simulink library "halin"  (R2021b)
settings: Solver=VariableStepAuto  StartTime=0.0  StopTime=10.0  RelTol=1e-3
undefined symbols (not defined in the file): KHAL_CAN1ABM1E2E_flg, KHAL_CAN1EPB1E2E_flg, KHAL_CAN1EPS1E2E_flg, KHAL_CAN1ESC1E2E_flg, KHAL_CAN1ESC5E2E_flg, KHAL_CAN3BMS1E2E_flg, KHAL_CAN3BMS6E2E_flg, KHAL_CAN3CCU1E2E_flg, KHAL_CAN3CCU2E2E_flg, KHAL_CAN3MCUBF1E2E_flg, KHAL_CAN3MCUBR1E2E_flg, KHAL_CAN3MCUNF1E2E_flg, KHAL_CAN3MCUNR1E2E_flg, KHAL_CAN3Shifter1E2E_flg, KHAL_CAN3Shifter2E2E_flg, KHAL_CAN6FCM2E2E_flg, KHAL_CAN6FCM4E2E_flg, TRUE
libraries: simulink x791, FVT_lib x214, hcu_lib x58
(part 23 of 25)

== system halin/HAL_IN/CAN3/MCU_N_R2/RrCoolanttempReqNidec ==
  Rr_CoolanttempReq_Nidec : Inport
  UnitConverter : DataTypeConversion  OutDataTypeStr=uint16
  convert_in : FVT_lib/hal/convert_in  gain=1  offset=-40
  VHAL_RrCoolanttempReqNidec_cnt : Outport
  wires:
  convert_in/1 -> VHAL_RrCoolanttempReqNidec_cnt/1
  UnitConverter/1 -> convert_in/1
  Rr_CoolanttempReq_Nidec/1 -> UnitConverter/1

== system halin/HAL_IN/CAN3/MCU_N_R2/RrEOPSpdSetNidec ==
  Rr_EOP_SpdSet_Nidec : Inport
  UnitConverter : DataTypeConversion  OutDataTypeStr=uint16
  VHAL_RrEOPSpdSetNidec_rpm : Outport
  wires:
  UnitConverter/1 -> VHAL_RrEOPSpdSetNidec_rpm/1
  Rr_EOP_SpdSet_Nidec/1 -> UnitConverter/1

== system halin/HAL_IN/CAN3/MCU_N_R2/RrFailcode1Nidec ==
  Rr_Failcode1_Nidec : Inport
  UnitConverter : DataTypeConversion  OutDataTypeStr=uint8
  VHAL_RrFailcode1Nidec_enum : Outport
  wires:
  UnitConverter/1 -> VHAL_RrFailcode1Nidec_enum/1
  Rr_Failcode1_Nidec/1 -> UnitConverter/1

== system halin/HAL_IN/CAN3/MCU_N_R2/RrFailcode2Nidec ==
  Rr_Failcode2_Nidec : Inport
  UnitConverter : DataTypeConversion  OutDataTypeStr=uint8
  VHAL_RrFailcode2Nidec_enum : Outport
  wires:
  UnitConverter/1 -> VHAL_RrFailcode2Nidec_enum/1
  Rr_Failcode2_Nidec/1 -> UnitConverter/1

== system halin/HAL_IN/CAN3/MCU_N_R2/RrFailcodehistory1Nidec ==
  Rr_Failcodehistory1_Nidec : Inport
  UnitConverter : DataTypeConversion  OutDataTypeStr=uint8
  VHAL_RrFailcodehistory1Nidec_enum : Outport
  wires:
  UnitConverter/1 -> VHAL_RrFailcodehistory1Nidec_enum/1
  Rr_Failcodehistory1_Nidec/1 -> UnitConverter/1

== system halin/HAL_IN/CAN3/MCU_N_R2/RrFailcodehistory2Nidec ==
  Rr_Failcodehistory2_Nidec : Inport
  UnitConverter : DataTypeConversion  OutDataTypeStr=uint8
  VHAL_RrFailcodehistory2Nidec_enum : Outport
  wires:
  UnitConverter/1 -> VHAL_RrFailcodehistory2Nidec_enum/1
  Rr_Failcodehistory2_Nidec/1 -> UnitConverter/1

== system halin/HAL_IN/CAN3/MCU_N_R2/RrLLCTempNidec ==
  Rr_LLCTemp_Nidec : Inport
  UnitConverter : DataTypeConversion  OutDataTypeStr=uint16
  convert_in : FVT_lib/hal/convert_in  gain=1  offset=-40
  VHAL_RrLLCTempNidec_C : Outport
  wires:
  convert_in/1 -> VHAL_RrLLCTempNidec_C/1
  UnitConverter/1 -> convert_in/1
  Rr_LLCTemp_Nidec/1 -> UnitConverter/1

== system halin/HAL_IN/CAN3/MCU_N_R2/RrLLCflowReqNidec ==
  Rr_LLCflowReq_Nidec : Inport
  UnitConverter : DataTypeConversion  OutDataTypeStr=uint8
  convert_in : FVT_lib/hal/convert_in  gain=0.25  offset=0
  VHAL_RrLLCflowReqNidec_Lpmin : Outport
  wires:
  convert_in/1 -> VHAL_RrLLCflowReqNidec_Lpmin/1
  UnitConverter/1 -> convert_in/1
  Rr_LLCflowReq_Nidec/1 -> UnitConverter/1

== system halin/HAL_IN/CAN3/MCU_N_R2/RrMCUTempWarnNidec ==
  Rr_MCUTempWarn_Nidec : Inport
  UnitConverter : DataTypeConversion  OutDataTypeStr=uint8
  VHAL_RrMCUTempWarnNidec_enum : Outport
  wires:
  UnitConverter/1 -> VHAL_RrMCUTempWarnNidec_enum/1
  Rr_MCUTempWarn_Nidec/1 -> UnitConverter/1

== system halin/HAL_IN/CAN3/MCU_N_R2/RrTMTempWarnNidec ==
  Rr_TMTempWarn_Nidec : Inport
  UnitConverter : DataTypeConversion  OutDataTypeStr=uint8
  VHAL_RrTMTempWarnNidec_enum : Outport
  wires:
  UnitConverter/1 -> VHAL_RrTMTempWarnNidec_enum/1
  Rr_TMTempWarn_Nidec/1 -> UnitConverter/1

== system halin/HAL_IN/CAN3/MCU_N_R3/RrMCU3HWVerNidec ==
  Rr_MCU3_HW_Ver_Nidec : Inport
  UnitConverter : DataTypeConversion  OutDataTypeStr=uint16
  VHAL_RrMCU3HWVerNidec_enum : Outport
  wires:
  UnitConverter/1 -> VHAL_RrMCU3HWVerNidec_enum/1
  Rr_MCU3_HW_Ver_Nidec/1 -> UnitConverter/1

== system halin/HAL_IN/CAN3/MCU_N_R3/RrMCU3SWVerNidec ==
  Rr_MCU3_SW_Ver_Nidec : Inport
  UnitConverter : DataTypeConversion  OutDataTypeStr=uint16
  VHAL_RrMCU3SWVerNidec_enum : Outport
  wires:
  UnitConverter/1 -> VHAL_RrMCU3SWVerNidec_enum/1
  Rr_MCU3_SW_Ver_Nidec/1 -> UnitConverter/1

== system halin/HAL_IN/CAN3/Shifter1/ShifterCRC8 ==
  Shifter_CRC8 : Inport
  UnitConverter : DataTypeConversion  OutDataTypeStr=uint8
  VHAL_ShifterCRC8_enum : Outport
  wires:
  UnitConverter/1 -> VHAL_ShifterCRC8_enum/1
  Shifter_CRC8/1 -> UnitConverter/1

== system halin/HAL_IN/CAN3/Shifter1/ShifterFailsta ==
  Shifter_Fail_sta : Inport
  UnitConverter : DataTypeConversion  OutDataTypeStr=uint8
  VHAL_ShifterFailsta_enum : Outport
  wires:
  UnitConverter/1 -> VHAL_ShifterFailsta_enum/1
  Shifter_Fail_sta/1 -> UnitConverter/1

== system halin/HAL_IN/CAN3/Shifter1/ShifterHandleCmd ==
  Shifter_Handle_Cmd : Inport
  UnitConverter : DataTypeConversion  OutDataTypeStr=uint8
  VHAL_ShifterHandleCmd_enum : Outport
  wires:
  UnitConverter/1 -> VHAL_ShifterHandleCmd_enum/1
  Shifter_Handle_Cmd/1 -> UnitConverter/1

== system halin/HAL_IN/CAN3/Shifter1/ShifterRC ==
  Shifter_RC : Inport
  UnitConverter : DataTypeConversion  OutDataTypeStr=uint8
  VHAL_ShifterRC_enum : Outport
  wires:
  UnitConverter/1 -> VHAL_ShifterRC_enum/1
  Shifter_RC/1 -> UnitConverter/1

== system halin/HAL_IN/CAN3/Shifter2/CSW2DimSwSta ==
  CSW2_DimSw_Sta : Inport
  UnitConverter : DataTypeConversion  OutDataTypeStr=uint8
  VHAL_CSW2DimSwSta_flg : Outport
  wires:
  UnitConverter/1 -> VHAL_CSW2DimSwSta_flg/1
  CSW2_DimSw_Sta/1 -> UnitConverter/1

== system halin/HAL_IN/CAN3/Shifter2/CSW2FWasSwSta ==
  CSW2_FWasSw_Sta : Inport
  UnitConverter : DataTypeConversion  OutDataTypeStr=uint8
  VHAL_CSW2FWasSwSta_enum : Outport
  wires:
  UnitConverter/1 -> VHAL_CSW2FWasSwSta_enum/1
  CSW2_FWasSw_Sta/1 -> UnitConverter/1

== system halin/HAL_IN/CAN3/Shifter2/CSW2FWipSwSta ==
  CSW2_FWipSw_Sta : Inport
  UnitConverter : DataTypeConversion  OutDataTypeStr=uint8
  VHAL_CSW2FWipSwSta_enum : Outport
  wires:
  UnitConverter/1 -> VHAL_CSW2FWipSwSta_enum/1
  CSW2_FWipSw_Sta/1 -> UnitConverter/1

== system halin/HAL_IN/CAN3/Shifter2/CSW2PassSWSta ==
  CSW2_PassSW_Sta : Inport
  UnitConverter : DataTypeConversion  OutDataTypeStr=uint8
  VHAL_CSW2PassSWSta_flg : Outport
  wires:
  UnitConverter/1 -> VHAL_CSW2PassSWSta_flg/1
  CSW2_PassSW_Sta/1 -> UnitConverter/1

== system halin/HAL_IN/CAN3/Shifter2/CSW2RWipWasSwSta ==
  CSW2_RWipWasSw_Sta : Inport
  UnitConverter : DataTypeConversion  OutDataTypeStr=uint8
  VHAL_CSW2RWipWasSwSta_enum : Outport
  wires:
  UnitConverter/1 -> VHAL_CSW2RWipWasSwSta_enum/1
  CSW2_RWipWasSw_Sta/1 -> UnitConverter/1

== system halin/HAL_IN/CAN3/Shifter2/CSW2TurnSwSta ==
  CSW2_TurnSw_Sta : Inport
  UnitConverter : DataTypeConversion  OutDataTypeStr=uint8
  VHAL_CSW2TurnSwSta_enum : Outport
  wires:
  UnitConverter/1 -> VHAL_CSW2TurnSwSta_enum/1
  CSW2_TurnSw_Sta/1 -> UnitConverter/1

== system halin/HAL_IN/CAN4/BodyZone_DR1/BDDSEATAntiSta ==
  BD_DSEAT_Anti_Sta : Inport
  UnitConverter : DataTypeConversion  OutDataTypeStr=uint8
  VHAL_BDDSEATAntiSta_flg : Outport
  wires:
  UnitConverter/1 -> VHAL_BDDSEATAntiSta_flg/1
  BD_DSEAT_Anti_Sta/1 -> UnitConverter/1

== system halin/HAL_IN/CAN4/BodyZone_DR1/BDDSEATEntryFunSta ==
  BD_DSEAT_EntryFun_Sta : Inport
  UnitConverter : DataTypeConversion  OutDataTypeStr=uint8
  VHAL_BDDSEATEntryFunSta_flg : Outport
  wires:
  UnitConverter/1 -> VHAL_BDDSEATEntryFunSta_flg/1
  BD_DSEAT_EntryFun_Sta/1 -> UnitConverter/1

== system halin/HAL_IN/CAN4/BodyZone_DR1/BDDSEATErrorSta ==
  BD_DSEAT_Error_Sta : Inport
  UnitConverter : DataTypeConversion  OutDataTypeStr=uint8
  VHAL_BDDSEATErrorSta_flg : Outport
  wires:
  UnitConverter/1 -> VHAL_BDDSEATErrorSta_flg/1
  BD_DSEAT_Error_Sta/1 -> UnitConverter/1

== system halin/HAL_IN/CAN4/BodyZone_DR1/BDDSEATMemSetSta ==
  BD_DSEAT_MemSet_Sta : Inport
  UnitConverter : DataTypeConversion  OutDataTypeStr=uint8
  VHAL_BDDSEATMemSetSta_enum : Outport
  wires:
  UnitConverter/1 -> VHAL_BDDSEATMemSetSta_enum/1
  BD_DSEAT_MemSet_Sta/1 -> UnitConverter/1

== system halin/HAL_IN/CAN4/BodyZone_DR1/BDDSEATModeSta ==
  BD_DSEAT_Mode_Sta : Inport
  UnitConverter : DataTypeConversion  OutDataTypeStr=uint8
  VHAL_BDDSEATModeSta_enum : Outport
  wires:
  UnitConverter/1 -> VHAL_BDDSEATModeSta_enum/1
  BD_DSEAT_Mode_Sta/1 -> UnitConverter/1

== system halin/HAL_IN/CAN4/BodyZone_DR1/BDDSEATVentSta ==
  BD_DSEAT_Vent_Sta : Inport
  UnitConverter : DataTypeConversion  OutDataTypeStr=uint8
  VHAL_BDDSEATVentSta_enum : Outport
  wires:
  UnitConverter/1 -> VHAL_BDDSEATVentSta_enum/1
  BD_DSEAT_Vent_Sta/1 -> UnitConverter/1

== system halin/HAL_IN/CAN4/BodyZone_DR1/BDDSEATheaterSta ==
  BD_DSEAT_heater_Sta : Inport
  UnitConverter : DataTypeConversion  OutDataTypeStr=uint8
  VHAL_BDDSEATheaterSta_enum : Outport
  wires:
  UnitConverter/1 -> VHAL_BDDSEATheaterSta_enum/1
  BD_DSEAT_heater_Sta/1 -> UnitConverter/1

== system halin/HAL_IN/CAN4/BodyZone_DR2/BDAPMWinFOpenedSta ==
  BD_APM_WinFOpened_Sta : Inport
  UnitConverter : DataTypeConversion  OutDataTypeStr=uint8
  VHAL_BDAPMWinFOpenedSta_pct : Outport
  wires:
  UnitConverter/1 -> VHAL_BDAPMWinFOpenedSta_pct/1
  BD_APM_WinFOpened_Sta/1 -> UnitConverter/1

== system halin/HAL_IN/CAN4/BodyZone_DR2/BDAPMWinROpenedSta ==
  BD_APM_WinROpened_Sta : Inport
  UnitConverter : DataTypeConversion  OutDataTypeStr=uint8
  VHAL_BDAPMWinROpenedSta_pct : Outport
  wires:
  UnitConverter/1 -> VHAL_BDAPMWinROpenedSta_pct/1
  BD_APM_WinROpened_Sta/1 -> UnitConverter/1

== system halin/HAL_IN/CAN4/BodyZone_DR2/BDDoorFHandleCloseSta ==
  BD_Door_FHandleClose_Sta : Inport
  UnitConverter : DataTypeConversion  OutDataTypeStr=uint8
  VHAL_BDDoorFHandleCloseSta_flg : Outport
  wires:
  UnitConverter/1 -> VHAL_BDDoorFHandleCloseSta_flg/1
  BD_Door_FHandleClose_Sta/1 -> UnitConverter/1

== system halin/HAL_IN/CAN4/BodyZone_DR2/BDDoorRHandleCloseSta ==
  BD_Door_RHandleClose_Sta : Inport
  UnitConverter : DataTypeConversion  OutDataTypeStr=uint8
  VHAL_BDDoorRHandleCloseSta_flg : Outport
  wires:
  UnitConverter/1 -> VHAL_BDDoorRHandleCloseSta_flg/1
  BD_Door_RHandleClose_Sta/1 -> UnitConverter/1

== system halin/HAL_IN/CAN4/BodyZone_PS1/BPPSEATErrorSta ==
  BP_PSEAT_Error_Sta : Inport
  UnitConverter : DataTypeConversion  OutDataTypeStr=uint8
  VHAL_BPPSEATErrorSta_flg : Outport
  wires:
  UnitConverter/1 -> VHAL_BPPSEATErrorSta_flg/1
  BP_PSEAT_Error_Sta/1 -> UnitConverter/1

== system halin/HAL_IN/CAN4/BodyZone_PS1/BPPSEATModeSta ==
  BP_PSEAT_Mode_Sta : Inport
  UnitConverter : DataTypeConversion  OutDataTypeStr=uint8
  VHAL_BPPSEATModeSta_enum : Outport
  wires:
  UnitConverter/1 -> VHAL_BPPSEATModeSta_enum/1
  BP_PSEAT_Mode_Sta/1 -> UnitConverter/1

== system halin/HAL_IN/CAN4/BodyZone_PS1/BPPSEATVentSta ==
  BP_PSEAT_Vent_Sta : Inport
  UnitConverter : DataTypeConversion  OutDataTypeStr=uint8
  VHAL_BPPSEATVentSta_enum : Outport
  wires:
  UnitConverter/1 -> VHAL_BPPSEATVentSta_enum/1
  BP_PSEAT_Vent_Sta/1 -> UnitConverter/1

== system halin/HAL_IN/CAN4/BodyZone_PS1/BPPSEATheaterSta ==
  BP_PSEAT_heater_Sta : Inport
  UnitConverter : DataTypeConversion  OutDataTypeStr=uint8
  VHAL_BPPSEATheaterSta_enum : Outport
  wires:
  UnitConverter/1 -> VHAL_BPPSEATheaterSta_enum/1
  BP_PSEAT_heater_Sta/1 -> UnitConverter/1

== system halin/HAL_IN/CAN4/BodyZone_PS1/BPPTGActiveSta ==
  BP_PTG_Active_Sta : Inport
  UnitConverter : DataTypeConversion  OutDataTypeStr=uint8
  VHAL_BPPTGActiveSta_enum : Outport
  wires:
  UnitConverter/1 -> VHAL_BPPTGActiveSta_enum/1
  BP_PTG_Active_Sta/1 -> UnitConverter/1

== system halin/HAL_IN/CAN4/BodyZone_PS1/BPPTGExistSta ==
  BP_PTG_Exist_Sta : Inport
  UnitConverter : DataTypeConversion  OutDataTypeStr=uint8
  VHAL_BPPTGExistSta_flg : Outport
  wires:
  UnitConverter/1 -> VHAL_BPPTGExistSta_flg/1
  BP_PTG_Exist_Sta/1 -> UnitConverter/1

== system halin/HAL_IN/CAN4/BodyZone_PS1/BPPTGInsideSW1Sta ==
  BP_PTG_InsideSW1_Sta : Inport
  UnitConverter : DataTypeConversion  OutDataTypeStr=uint8
  VHAL_BPPTGInsideSW1Sta_enum : Outport
  wires:
  UnitConverter/1 -> VHAL_BPPTGInsideSW1Sta_enum/1
  BP_PTG_InsideSW1_Sta/1 -> UnitConverter/1

== system halin/HAL_IN/CAN4/BodyZone_PS1/BPPTGInsideSW2Sta ==
  BP_PTG_InsideSW2_Sta : Inport
  UnitConverter : DataTypeConversion  OutDataTypeStr=uint8
  VHAL_BPPTGInsideSW2Sta_enum : Outport
  wires:
  UnitConverter/1 -> VHAL_BPPTGInsideSW2Sta_enum/1
  BP_PTG_InsideSW2_Sta/1 -> UnitConverter/1

== system halin/HAL_IN/CAN4/BodyZone_PS1/BPPTGIsSetHeightSta ==
  BP_PTG_IsSetHeight_Sta : Inport
  UnitConverter : DataTypeConversion  OutDataTypeStr=uint8
  VHAL_BPPTGIsSetHeightSta_flg : Outport
  wires:
  UnitConverter/1 -> VHAL_BPPTGIsSetHeightSta_flg/1
  BP_PTG_IsSetHeight_Sta/1 -> UnitConverter/1

== system halin/HAL_IN/CAN4/BodyZone_PS1/BPPTGLeftHallPosnSta ==
  BP_PTG_LeftHallPosn_Sta : Inport
  UnitConverter : DataTypeConversion  OutDataTypeStr=uint16
  VHAL_BPPTGLeftHallPosnSta_enum : Outport
  wires:
  UnitConverter/1 -> VHAL_BPPTGLeftHallPosnSta_enum/1
  BP_PTG_LeftHallPosn_Sta/1 -> UnitConverter/1

== system halin/HAL_IN/CAN4/BodyZone_PS1/BPPTGOpenRatioSta ==
  BP_PTG_OpenRatio_Sta : Inport
  UnitConverter : DataTypeConversion  OutDataTypeStr=uint8
  VHAL_BPPTGOpenRatioSta_pct : Outport
  wires:
  UnitConverter/1 -> VHAL_BPPTGOpenRatioSta_pct/1
  BP_PTG_OpenRatio_Sta/1 -> UnitConverter/1

== system halin/HAL_IN/CAN4/BodyZone_PS1/BPPTGRDILCmd ==
  BP_PTG_RDIL_Cmd : Inport
  UnitConverter : DataTypeConversion  OutDataTypeStr=uint8
  VHAL_BPPTGRDILCmd_enum : Outport
  wires:
  UnitConverter/1 -> VHAL_BPPTGRDILCmd_enum/1
  BP_PTG_RDIL_Cmd/1 -> UnitConverter/1

== system halin/HAL_IN/CAN4/BodyZone_PS1/BPPTGSysSta ==
  BP_PTG_Sys_Sta : Inport
  UnitConverter : DataTypeConversion  OutDataTypeStr=uint8
  VHAL_BPPTGSysSta_enum : Outport
  wires:
  UnitConverter/1 -> VHAL_BPPTGSysSta_enum/1
  BP_PTG_Sys_Sta/1 -> UnitConverter/1

== system halin/HAL_IN/CAN4/BodyZone_PS2/BPAPMWinFOpenedSta ==
  BP_APM_WinFOpened_Sta : Inport
  UnitConverter : DataTypeConversion  OutDataTypeStr=uint8
  VHAL_BPAPMWinFOpenedSta_pct : Outport
  wires:
  UnitConverter/1 -> VHAL_BPAPMWinFOpenedSta_pct/1
  BP_APM_WinFOpened_Sta/1 -> UnitConverter/1

== system halin/HAL_IN/CAN4/BodyZone_PS2/BPAPMWinROpenedSta ==
  BP_APM_WinROpened_Sta : Inport
  UnitConverter : DataTypeConversion  OutDataTypeStr=uint8
  VHAL_BPAPMWinROpenedSta_pct : Outport
  wires:
  UnitConverter/1 -> VHAL_BPAPMWinROpenedSta_pct/1
  BP_APM_WinROpened_Sta/1 -> UnitConverter/1

== system halin/HAL_IN/CAN4/BodyZone_PS2/BPDoorFHandleCloseSta ==
  BP_Door_FHandleClose_Sta : Inport
  UnitConverter : DataTypeConversion  OutDataTypeStr=uint8
  VHAL_BPDoorFHandleCloseSta_flg : Outport
  wires:
  UnitConverter/1 -> VHAL_BPDoorFHandleCloseSta_flg/1
  BP_Door_FHandleClose_Sta/1 -> UnitConverter/1

== system halin/HAL_IN/CAN4/BodyZone_PS2/BPDoorRHandleCloseSta ==
  BP_Door_RHandleClose_Sta : Inport
  UnitConverter : DataTypeConversion  OutDataTypeStr=uint8
  VHAL_BPDoorRHandleCloseSta_flg : Outport
  wires:
  UnitConverter/1 -> VHAL_BPDoorRHandleCloseSta_flg/1
  BP_Door_RHandleClose_Sta/1 -> UnitConverter/1

== system halin/HAL_IN/CAN4/BodyZone_PS2/BPSEATLVentSta ==
  BP_SEAT_LVent_Sta : Inport
  UnitConverter : DataTypeConversion  OutDataTypeStr=uint8
  VHAL_BPSEATLVentSta_enum : Outport
  wires:
  UnitConverter/1 -> VHAL_BPSEATLVentSta_enum/1
  BP_SEAT_LVent_Sta/1 -> UnitConverter/1

== system halin/HAL_IN/CAN4/BodyZone_PS2/BPSEATMLVentSta ==
  BP_SEAT_MLVent_Sta : Inport
  UnitConverter : DataTypeConversion  OutDataTypeStr=uint8
  VHAL_BPSEATMLVentSta_enum : Outport
  wires:
  UnitConverter/1 -> VHAL_BPSEATMLVentSta_enum/1
  BP_SEAT_MLVent_Sta/1 -> UnitConverter/1

== system halin/HAL_IN/CAN4/BodyZone_PS2/BPSEATMRVentSta ==
  BP_SEAT_MRVent_Sta : Inport
  UnitConverter : DataTypeConversion  OutDataTypeStr=uint8
  VHAL_BPSEATMRVentSta_enum : Outport
  wires:
  UnitConverter/1 -> VHAL_BPSEATMRVentSta_enum/1
  BP_SEAT_MRVent_Sta/1 -> UnitConverter/1

== system halin/HAL_IN/CAN4/BodyZone_PS2/BPSEATRVentSta ==
  BP_SEAT_RVent_Sta : Inport
  UnitConverter : DataTypeConversion  OutDataTypeStr=uint8
  VHAL_BPSEATRVentSta_enum : Outport
  wires:
  UnitConverter/1 -> VHAL_BPSEATRVentSta_enum/1
  BP_SEAT_RVent_Sta/1 -> UnitConverter/1

== system halin/HAL_IN/CAN4/DKC1/DKCKeyNumSta ==
  DKC_KeyNum_Sta : Inport
  UnitConverter : DataTypeConversion  OutDataTypeStr=uint8
  VHAL_DKCKeyNumSta_enum : Outport
  wires:
  UnitConverter/1 -> VHAL_DKCKeyNumSta_enum/1
  DKC_KeyNum_Sta/1 -> UnitConverter/1

== system halin/HAL_IN/CAN4/DKC1/DKCKeyTypeSta ==
  DKC_KeyType_Sta : Inport
  UnitConverter : DataTypeConversion  OutDataTypeStr=uint8
  VHAL_DKCKeyTypeSta_enum : Outport
  wires:
  UnitConverter/1 -> VHAL_DKCKeyTypeSta_enum/1
  DKC_KeyType_Sta/1 -> UnitConverter/1

== system halin/HAL_IN/CAN4/DKC1/DKCPDkeyAreaRAPSSta ==
  DKC_PDkeyAreaRAPS_Sta : Inport
  UnitConverter : DataTypeConversion  OutDataTypeStr=uint8
  VHAL_DKCPDkeyAreaRAPSSta_enum : Outport
  wires:
  UnitConverter/1 -> VHAL_DKCPDkeyAreaRAPSSta_enum/1
  DKC_PDkeyAreaRAPS_Sta/1 -> UnitConverter/1

== system halin/HAL_IN/CAN4/DKC1/DKCParkingModeCmd ==
  DKC_ParkingMode_Cmd : Inport
  UnitConverter : DataTypeConversion  OutDataTypeStr=uint8
  VHAL_DKCParkingModeCmd_enum : Outport
  wires:
  UnitConverter/1 -> VHAL_DKCParkingModeCmd_enum/1
  DKC_ParkingMode_Cmd/1 -> UnitConverter/1

== system halin/HAL_IN/CAN4/DKC1/DKCReVehData ==
  DKC_Re_VehData : Inport
  UnitConverter : DataTypeConversion  OutDataTypeStr=uint8
  VHAL_DKCReVehData_enum : Outport
  wires:
  UnitConverter/1 -> VHAL_DKCReVehData_enum/1
  DKC_Re_VehData/1 -> UnitConverter/1

== system halin/HAL_IN/CAN4/DKC1/PCommandToBCM ==
  P_CommandToBCM : Inport
  UnitConverter : DataTypeConversion  OutDataTypeStr=uint8
  VHAL_PCommandToBCM_enum : Outport
  wires:
  UnitConverter/1 -> VHAL_PCommandToBCM_enum/1
  P_CommandToBCM/1 -> UnitConverter/1

== system halin/HAL_IN/CAN4/DKC1/PCommandToPTG ==
  P_CommandToPTG : Inport
  UnitConverter : DataTypeConversion  OutDataTypeStr=uint8
  VHAL_PCommandToPTG_enum : Outport
  wires:
  UnitConverter/1 -> VHAL_PCommandToPTG_enum/1
  P_CommandToPTG/1 -> UnitConverter/1

== system halin/HAL_IN/CAN4/DKC1/PDKeyAreaLockUnlock ==
  P_DKey_Area_LockUnlock : Inport
  UnitConverter : DataTypeConversion  OutDataTypeStr=uint8
  VHAL_PDKeyAreaLockUnlock_enum : Outport
  wires:
  UnitConverter/1 -> VHAL_PDKeyAreaLockUnlock_enum/1
  P_DKey_Area_LockUnlock/1 -> UnitConverter/1

== system halin/HAL_IN/CAN4/DKC1/PDKeyAreaPS ==
  P_DKey_Area_PS : Inport
  UnitConverter : DataTypeConversion  OutDataTypeStr=uint8
  VHAL_PDKeyAreaPS_enum : Outport
  wires:
  UnitConverter/1 -> VHAL_PDKeyAreaPS_enum/1
  P_DKey_Area_PS/1 -> UnitConverter/1

== system halin/HAL_IN/CAN4/DKC1/PDKeyAreaPTG ==
  P_DKey_Area_PTG : Inport
  UnitConverter : DataTypeConversion  OutDataTypeStr=uint8
  VHAL_PDKeyAreaPTG_enum : Outport
  wires:
  UnitConverter/1 -> VHAL_PDKeyAreaPTG_enum/1
  P_DKey_Area_PTG/1 -> UnitConverter/1

== system halin/HAL_IN/CAN4/DKC1/PDKeyWelcome ==
  P_DKey_Welcome : Inport
  UnitConverter : DataTypeConversion  OutDataTypeStr=uint8
  VHAL_PDKeyWelcome_enum : Outport
  wires:
  UnitConverter/1 -> VHAL_PDKeyWelcome_enum/1
  P_DKey_Welcome/1 -> UnitConverter/1

== system halin/HAL_IN/CAN4/DKC1/PDkeyShowIVI ==
  P_Dkey_Show_IVI : Inport
  UnitConverter : DataTypeConversion  OutDataTypeStr=uint8
  VHAL_PDkeyShowIVI_enum : Outport
  wires:
  UnitConverter/1 -> VHAL_PDkeyShowIVI_enum/1
  P_Dkey_Show_IVI/1 -> UnitConverter/1

== system halin/HAL_IN/CAN4/DKC1/PKeyMiss ==
  P_KeyMiss : Inport
  UnitConverter : DataTypeConversion  OutDataTypeStr=uint8
  VHAL_PKeyMiss_flg : Outport
  wires:
  UnitConverter/1 -> VHAL_PKeyMiss_flg/1
  P_KeyMiss/1 -> UnitConverter/1

== system halin/HAL_IN/CAN4/DKC1/PKeyMode ==
  P_KeyMode : Inport
  UnitConverter : DataTypeConversion  OutDataTypeStr=uint8
  VHAL_PKeyMode_enum : Outport
  wires:
  UnitConverter/1 -> VHAL_PKeyMode_enum/1
  P_KeyMode/1 -> UnitConverter/1

== system halin/HAL_IN/CAN4/DKC1/PUIDLowPower ==
  P_UID_LowPower : Inport
  UnitConverter : DataTypeConversion  OutDataTypeStr=uint8
  VHAL_PUIDLowPower_flg : Outport
  wires:
  UnitConverter/1 -> VHAL_PUIDLowPower_flg/1
  P_UID_LowPower/1 -> UnitConverter/1

== system halin/HAL_IN/CAN4/DKC2/EncryptionDATA063 ==
  EncryptionDATA_0_63 : Inport
  UnitConverter : DataTypeConversion  OutDataTypeStr=uint64
  VHAL_EncryptionDATA063_enum : Outport
  wires:
  UnitConverter/1 -> VHAL_EncryptionDATA063_enum/1
  EncryptionDATA_0_63/1 -> UnitConverter/1

== system halin/HAL_IN/CAN4/DKC2/EncryptionDATA64127 ==
  EncryptionDATA_64_127 : Inport
  UnitConverter : DataTypeConversion  OutDataTypeStr=uint64
  VHAL_EncryptionDATA64127_enum : Outport
  wires:
  UnitConverter/1 -> VHAL_EncryptionDATA64127_enum/1
  EncryptionDATA_64_127/1 -> UnitConverter/1

== system halin/HAL_IN/CAN4/DKC2/RandomNumberX ==
  Random_Number_X : Inport
  UnitConverter : DataTypeConversion  OutDataTypeStr=uint64
  VHAL_RandomNumberX_enum : Outport
  wires:
  UnitConverter/1 -> VHAL_RandomNumberX_enum/1
  Random_Number_X/1 -> UnitConverter/1

== system halin/HAL_IN/CAN4/PTG1/PTGActiveSta ==
  PTG_Active_Sta : Inport
  UnitConverter : DataTypeConversion  OutDataTypeStr=uint8
  VHAL_PTGActiveSta_enum : Outport
  wires:
  UnitConverter/1 -> VHAL_PTGActiveSta_enum/1
  PTG_Active_Sta/1 -> UnitConverter/1

== system halin/HAL_IN/CAN4/PTG1/PTGAutoStaus ==
  PTG_AutoStaus : Inport
  UnitConverter : DataTypeConversion  OutDataTypeStr=uint8
  VHAL_PTGAutoStaus_flg : Outport
  wires:
  UnitConverter/1 -> VHAL_PTGAutoStaus_flg/1
  PTG_AutoStaus/1 -> UnitConverter/1

== system halin/HAL_IN/CAN4/PTG1/PTGExist ==
  PTG_Exist : Inport
  UnitConverter : DataTypeConversion  OutDataTypeStr=uint8
  VHAL_PTGExist_flg : Outport
  wires:
  UnitConverter/1 -> VHAL_PTGExist_flg/1
  PTG_Exist/1 -> UnitConverter/1

== system halin/HAL_IN/CAN4/PTG1/PTGHWVer ==
  PTG_HW_Ver : Inport
  UnitConverter : DataTypeConversion  OutDataTypeStr=uint8
  VHAL_PTGHWVer_enum : Outport
  wires:
  UnitConverter/1 -> VHAL_PTGHWVer_enum/1
  PTG_HW_Ver/1 -> UnitConverter/1

== system halin/HAL_IN/CAN4/PTG1/PTGInnerSW2 ==
  PTG_Inner_SW_2 : Inport
  UnitConverter : DataTypeConversion  OutDataTypeStr=uint8
  VHAL_PTGInnerSW2_enum : Outport
  wires:
  UnitConverter/1 -> VHAL_PTGInnerSW2_enum/1
  PTG_Inner_SW_2/1 -> UnitConverter/1

== system halin/HAL_IN/CAN4/PTG1/PTGIsSetHeight ==
  PTG_Is_Set_Height : Inport
  UnitConverter : DataTypeConversion  OutDataTypeStr=uint8
  VHAL_PTGIsSetHeight_flg : Outport
  wires:
  UnitConverter/1 -> VHAL_PTGIsSetHeight_flg/1
  PTG_Is_Set_Height/1 -> UnitConverter/1

== system halin/HAL_IN/CAN4/PTG1/PTGOpenRatio ==
  PTG_Open_Ratio : Inport
  UnitConverter : DataTypeConversion  OutDataTypeStr=uint8
  VHAL_PTGOpenRatio_pct : Outport
  wires:
  UnitConverter/1 -> VHAL_PTGOpenRatio_pct/1
  PTG_Open_Ratio/1 -> UnitConverter/1

== system halin/HAL_IN/CAN4/PTG1/PTGRDILSta ==
  PTG_RDIL_Sta : Inport
  UnitConverter : DataTypeConversion  OutDataTypeStr=uint8
  VHAL_PTGRDILSta_enum : Outport
  wires:
  UnitConverter/1 -> VHAL_PTGRDILSta_enum/1
  PTG_RDIL_Sta/1 -> UnitConverter/1

== system halin/HAL_IN/CAN4/PTG1/PTGSWVer ==
  PTG_SW_Ver : Inport
  UnitConverter : DataTypeConversion  OutDataTypeStr=uint8
  VHAL_PTGSWVer_enum : Outport
  wires:
  UnitConverter/1 -> VHAL_PTGSWVer_enum/1
  PTG_SW_Ver/1 -> UnitConverter/1

== system halin/HAL_IN/CAN4/PTG1/PTGSysSta ==
  PTG_Sys_Sta : Inport
  UnitConverter : DataTypeConversion  OutDataTypeStr=uint8
  VHAL_PTGSysSta_enum : Outport
  wires:
  UnitConverter/1 -> VHAL_PTGSysSta_enum/1
  PTG_Sys_Sta/1 -> UnitConverter/1

== system halin/HAL_IN/CAN4/ZONE_DR1/DrLockSta ==
  DrLockSta : Inport
  UnitConverter : DataTypeConversion  OutDataTypeStr=uint8
  VHAL_DrLockSta_flg : Outport
  wires:
  UnitConverter/1 -> VHAL_DrLockSta_flg/1
  DrLockSta/1 -> UnitConverter/1

== system halin/HAL_IN/CAN4/ZONE_DR1/MIRRORFOLDSW ==
  MIRROR_FOLD_SW : Inport
  UnitConverter : DataTypeConversion  OutDataTypeStr=uint8
  VHAL_MIRRORFOLDSW_flg : Outport
  wires:
  UnitConverter/1 -> VHAL_MIRRORFOLDSW_flg/1
  MIRROR_FOLD_SW/1 -> UnitConverter/1

== system halin/HAL_IN/CAN4/ZONE_DR1/RLTurnLPErr ==
  RLTurnLPErr : Inport
  UnitConverter : DataTypeConversion  OutDataTypeStr=uint8
  VHAL_RLTurnLPErr_flg : Outport
  wires:
  UnitConverter/1 -> VHAL_RLTurnLPErr_flg/1
  RLTurnLPErr/1 -> UnitConverter/1

== system halin/HAL_IN/CAN4/ZONE_DR1/RLTurnLampC ==
  RLTurnLampC : Inport
  UnitConverter : DataTypeConversion  OutDataTypeStr=uint8
  convert_in : FVT_lib/hal/convert_in  gain=10  offset=0
  VHAL_RLTurnLampC_mA : Outport
  wires:
  convert_in/1 -> VHAL_RLTurnLampC_mA/1
  UnitConverter/1 -> convert_in/1
  RLTurnLampC/1 -> UnitConverter/1

== system halin/HAL_IN/CAN4/ZONE_DR1/RRTurnLPErr ==
  RRTurnLPErr : Inport
  UnitConverter : DataTypeConversion  OutDataTypeStr=uint8
  VHAL_RRTurnLPErr_flg : Outport
  wires:
  UnitConverter/1 -> VHAL_RRTurnLPErr_flg/1
  RRTurnLPErr/1 -> UnitConverter/1

== system halin/HAL_IN/CAN4/ZONE_DR1/RRTurnLampC ==
  RRTurnLampC : Inport
  UnitConverter : DataTypeConversion  OutDataTypeStr=uint8
  convert_in : FVT_lib/hal/convert_in  gain=10  offset=0
  VHAL_RRTurnLampC_mA : Outport
  wires:
  convert_in/1 -> VHAL_RRTurnLampC_mA/1
  UnitConverter/1 -> convert_in/1
  RRTurnLampC/1 -> UnitConverter/1

== system halin/HAL_IN/CAN4/ZONE_DR1/RWiperAS ==
  RWiperAS : Inport
  UnitConverter : DataTypeConversion  OutDataTypeStr=uint8
  VHAL_RWiperAS_flg : Outport
  wires:
  UnitConverter/1 -> VHAL_RWiperAS_flg/1
  RWiperAS/1 -> UnitConverter/1

== system halin/HAL_IN/CAN4/ZONE_DR1/RWiperProtection ==
  RWiperProtection : Inport
  UnitConverter : DataTypeConversion  OutDataTypeStr=uint8
  VHAL_RWiperProtection_flg : Outport
  wires:
  UnitConverter/1 -> VHAL_RWiperProtection_flg/1
  RWiperProtection/1 -> UnitConverter/1

== system halin/HAL_IN/CAN4/ZONE_DR_VCU/BlowerErr ==
  Blower_Err : Inport
  UnitConverter : DataTypeConversion  OutDataTypeStr=uint8
  VHAL_BlowerErr_enum : Outport
  wires:
  UnitConverter/1 -> VHAL_BlowerErr_enum/1
  Blower_Err/1 -> UnitConverter/1

== system halin/HAL_IN/CAN4/ZONE_DR_VCU/DrPMMLVOutPErrLmp ==
  DrPMMLVOutPErrLmp : Inport
  UnitConverter : DataTypeConversion  OutDataTypeStr=uint8
  VHAL_DrPMMLVOutPErrLmp_flg : Outport
  wires:
  UnitConverter/1 -> VHAL_DrPMMLVOutPErrLmp_flg/1
  DrPMMLVOutPErrLmp/1 -> UnitConverter/1

== system halin/HAL_IN/CAN4/ZONE_DR_VCU/DrPMMSysErrLmp ==
  DrPMMSysErrLmp : Inport
  UnitConverter : DataTypeConversion  OutDataTypeStr=uint8
  VHAL_DrPMMSysErrLmp_flg : Outport
  wires:
  UnitConverter/1 -> VHAL_DrPMMSysErrLmp_flg/1
  DrPMMSysErrLmp/1 -> UnitConverter/1

== system halin/HAL_IN/CAN4/ZONE_DR_VCU/DrSCPSysErrLmp ==
  DrSCPSysErrLmp : Inport
  UnitConverter : DataTypeConversion  OutDataTypeStr=uint8
  VHAL_DrSCPSysErrLmp_flg : Outport
  wires:
  UnitConverter/1 -> VHAL_DrSCPSysErrLmp_flg/1
  DrSCPSysErrLmp/1 -> UnitConverter/1

== system halin/HAL_IN/CAN4/ZONE_DR_VCU/DrStdAErrSta ==
  DrStdAErrSta : Inport
  UnitConverter : DataTypeConversion  OutDataTypeStr=uint8
  VHAL_DrStdAErrSta_flg : Outport
  wires:
  UnitConverter/1 -> VHAL_DrStdAErrSta_flg/1
  DrStdAErrSta/1 -> UnitConverter/1

== system halin/HAL_IN/CAN4/ZONE_DR_VCU/LeftHallPos ==
  LeftHall_Pos : Inport
  UnitConverter : DataTypeConversion  OutDataTypeStr=uint16
  VHAL_LeftHallPos_enum : Outport
  wires:
  UnitConverter/1 -> VHAL_LeftHallPos_enum/1
  LeftHall_Pos/1 -> UnitConverter/1

== system halin/HAL_IN/CAN4/ZONE_DR_VCU/SolarL ==
  SolarL : Inport
  UnitConverter : DataTypeConversion  OutDataTypeStr=uint8
  convert_in : FVT_lib/hal/convert_in  gain=5  offset=0
  VHAL_SolarL_W : Outport
  wires:
  convert_in/1 -> VHAL_SolarL_W/1
  UnitConverter/1 -> convert_in/1
  SolarL/1 -> UnitConverter/1

== system halin/HAL_IN/CAN4/ZONE_DR_VCU/SolarLErr ==
  SolarL_Err : Inport
  UnitConverter : DataTypeConversion  OutDataTypeStr=uint8
  VHAL_SolarLErr_enum : Outport
  wires:
  UnitConverter/1 -> VHAL_SolarLErr_enum/1
  SolarL_Err/1 -> UnitConverter/1

== system halin/HAL_IN/CAN4/ZONE_DR_VCU/SolarR ==
  SolarR : Inport
  UnitConverter : DataTypeConversion  OutDataTypeStr=uint8
  convert_in : FVT_lib/hal/convert_in  gain=5  offset=0
  VHAL_SolarR_W : Outport
  wires:
  convert_in/1 -> VHAL_SolarR_W/1
  UnitConverter/1 -> convert_in/1
  SolarR/1 -> UnitConverter/1

== system halin/HAL_IN/CAN4/ZONE_DR_VCU/SolarRErr ==
  SolarR_Err : Inport
  UnitConverter : DataTypeConversion  OutDataTypeStr=uint8
  VHAL_SolarRErr_enum : Outport
  wires:
  UnitConverter/1 -> VHAL_SolarRErr_enum/1
  SolarR_Err/1 -> UnitConverter/1

== system halin/HAL_IN/CAN4/ZONE_DR_VCU/TFaceL ==
  T_Face_L : Inport
  UnitConverter : DataTypeConversion  OutDataTypeStr=uint8
  convert_in : FVT_lib/hal/convert_in  gain=0.5  offset=-40
  VHAL_TFaceL_C : Outport
  wires:
  convert_in/1 -> VHAL_TFaceL_C/1
  UnitConverter/1 -> convert_in/1
  T_Face_L/1 -> UnitConverter/1

== system halin/HAL_IN/CAN4/ZONE_DR_VCU/TFaceLErr ==
  T_Face_L_Err : Inport
  UnitConverter : DataTypeConversion  OutDataTypeStr=uint8
  VHAL_TFaceLErr_enum : Outport
  wires:
  UnitConverter/1 -> VHAL_TFaceLErr_enum/1
  T_Face_L_Err/1 -> UnitConverter/1

== system halin/HAL_IN/CAN4/ZONE_DR_VCU/TFaceR ==
  T_Face_R : Inport
  UnitConverter : DataTypeConversion  OutDataTypeStr=uint8
  convert_in : FVT_lib/hal/convert_in  gain=0.5  offset=-40
  VHAL_TFaceR_C : Outport
  wires:
  convert_in/1 -> VHAL_TFaceR_C/1
  UnitConverter/1 -> convert_in/1
  T_Face_R/1 -> UnitConverter/1

== system halin/HAL_IN/CAN4/ZONE_DR_VCU/TFaceRErr ==
  T_Face_R_Err : Inport
  UnitConverter : DataTypeConversion  OutDataTypeStr=uint8
  VHAL_TFaceRErr_enum : Outport
  wires:
  UnitConverter/1 -> VHAL_TFaceRErr_enum/1
  T_Face_R_Err/1 -> UnitConverter/1

== system halin/HAL_IN/CAN4/ZONE_DR_VCU/TFaceRr ==
  T_Face_Rr : Inport
  UnitConverter : DataTypeConversion  OutDataTypeStr=uint8
  convert_in : FVT_lib/hal/convert_in  gain=0.5  offset=-40
  VHAL_TFaceRr_C : Outport
  wires:
  convert_in/1 -> VHAL_TFaceRr_C/1
  UnitConverter/1 -> convert_in/1
  T_Face_Rr/1 -> UnitConverter/1

== system halin/HAL_IN/CAN4/ZONE_DR_VCU/TFaceRrErr ==
  T_Face_Rr_Err : Inport
  UnitConverter : DataTypeConversion  OutDataTypeStr=uint8
  VHAL_TFaceRrErr_enum : Outport
  wires:
  UnitConverter/1 -> VHAL_TFaceRrErr_enum/1
  T_Face_Rr_Err/1 -> UnitConverter/1

== system halin/HAL_IN/CAN4/ZONE_DR_VCU/TFootL ==
  T_Foot_L : Inport
  UnitConverter : DataTypeConversion  OutDataTypeStr=uint8
  convert_in : FVT_lib/hal/convert_in  gain=0.5  offset=-40
  VHAL_TFootL_C : Outport
  wires:
  convert_in/1 -> VHAL_TFootL_C/1
  UnitConverter/1 -> convert_in/1
  T_Foot_L/1 -> UnitConverter/1

== system halin/HAL_IN/CAN4/ZONE_DR_VCU/TFootLErr ==
  T_Foot_L_Err : Inport
  UnitConverter : DataTypeConversion  OutDataTypeStr=uint8
  VHAL_TFootLErr_enum : Outport
  wires:
  UnitConverter/1 -> VHAL_TFootLErr_enum/1
  T_Foot_L_Err/1 -> UnitConverter/1

== system halin/HAL_IN/CAN4/ZONE_DR_VCU/TFootR ==
  T_Foot_R : Inport
  UnitConverter : DataTypeConversion  OutDataTypeStr=uint8
  convert_in : FVT_lib/hal/convert_in  gain=0.5  offset=-40
  VHAL_TFootR_C : Outport
  wires:
  convert_in/1 -> VHAL_TFootR_C/1
  UnitConverter/1 -> convert_in/1
  T_Foot_R/1 -> UnitConverter/1

== system halin/HAL_IN/CAN4/ZONE_DR_VCU/TFootRErr ==
  T_Foot_R_Err : Inport
  UnitConverter : DataTypeConversion  OutDataTypeStr=uint8
  VHAL_TFootRErr_enum : Outport
  wires:
  UnitConverter/1 -> VHAL_TFootRErr_enum/1
  T_Foot_R_Err/1 -> UnitConverter/1

== system halin/HAL_IN/CAN4/ZONE_DR_VCU/TFootRr ==
  T_Foot_Rr : Inport
  UnitConverter : DataTypeConversion  OutDataTypeStr=uint8
  convert_in : FVT_lib/hal/convert_in  gain=0.5  offset=-40
  VHAL_TFootRr_C : Outport
  wires:
  convert_in/1 -> VHAL_TFootRr_C/1
  UnitConverter/1 -> convert_in/1
  T_Foot_Rr/1 -> UnitConverter/1

== system halin/HAL_IN/CAN4/ZONE_DR_VCU/TFootRrErr ==
  T_Foot_Rr_Err : Inport
  UnitConverter : DataTypeConversion  OutDataTypeStr=uint8
  VHAL_TFootRrErr_enum : Outport
  wires:
  UnitConverter/1 -> VHAL_TFootRrErr_enum/1
  T_Foot_Rr_Err/1 -> UnitConverter/1

== system halin/HAL_IN/CAN4/ZONE_DR_VCU/Tevap ==
  Tevap : Inport
  UnitConverter : DataTypeConversion  OutDataTypeStr=uint8
  convert_in : FVT_lib/hal/convert_in  gain=0.5  offset=-40
  VHAL_Tevap_C : Outport
  wires:
  convert_in/1 -> VHAL_Tevap_C/1
  UnitConverter/1 -> convert_in/1
  Tevap/1 -> UnitConverter/1

== system halin/HAL_IN/CAN4/ZONE_DR_VCU/TevapErr ==
  Tevap_Err : Inport
  UnitConverter : DataTypeConversion  OutDataTypeStr=uint8
  VHAL_TevapErr_enum : Outport
  wires:
  UnitConverter/1 -> VHAL_TevapErr_enum/1
  Tevap_Err/1 -> UnitConverter/1

== system halin/HAL_IN/CAN4/ZONE_DR_VCU/Tincar ==
  Tincar : Inport
  UnitConverter : DataTypeConversion  OutDataTypeStr=uint8
  convert_in : FVT_lib/hal/convert_in  gain=0.5  offset=-40
  VHAL_Tincar_C : Outport
  wires:
  convert_in/1 -> VHAL_Tincar_C/1
  UnitConverter/1 -> convert_in/1
  Tincar/1 -> UnitConverter/1

== system halin/HAL_IN/CAN4/ZONE_DR_VCU/TincarErr ==
  Tincar_Err : Inport
  UnitConverter : DataTypeConversion  OutDataTypeStr=uint8
  VHAL_TincarErr_enum : Outport
  wires:
  UnitConverter/1 -> VHAL_TincarErr_enum/1
  Tincar_Err/1 -> UnitConverter/1

== system halin/HAL_IN/CAN4/ZONE_DR_VCU/ZoneDrMalfunLevel ==
  ZoneDrMalfunLevel : Inport
  UnitConverter : DataTypeConversion  OutDataTypeStr=uint8
  VHAL_ZoneDrMalfunLevel_enum : Outport
  wires:
  UnitConverter/1 -> VHAL_ZoneDrMalfunLevel_enum/1
  ZoneDrMalfunLevel/1 -> UnitConverter/1

== system halin/HAL_IN/CAN4/ZONE_FR1/ChargeInletLockSta ==
  ChargeInletLockSta : Inport
  UnitConverter : DataTypeConversion  OutDataTypeStr=uint8
  VHAL_ChargeInletLockSta_flg : Outport
  wires:
  UnitConverter/1 -> VHAL_ChargeInletLockSta_flg/1
  ChargeInletLockSta/1 -> UnitConverter/1

== system halin/HAL_IN/CAN4/ZONE_FR1/CompProEN ==
  CompProEN : Inport
  UnitConverter : DataTypeConversion  OutDataTypeStr=uint8
  VHAL_CompProEN_flg : Outport
  wires:
  UnitConverter/1 -> VHAL_CompProEN_flg/1
  CompProEN/1 -> UnitConverter/1

== system halin/HAL_IN/CAN4/ZONE_FR1/FLTurnLPErr ==
  FLTurnLPErr : Inport
  UnitConverter : DataTypeConversion  OutDataTypeStr=uint8
  VHAL_FLTurnLPErr_flg : Outport
  wires:
  UnitConverter/1 -> VHAL_FLTurnLPErr_flg/1
  FLTurnLPErr/1 -> UnitConverter/1

== system halin/HAL_IN/CAN4/ZONE_FR1/FLTurnLampC ==
  FLTurnLampC : Inport
  UnitConverter : DataTypeConversion  OutDataTypeStr=uint8
  convert_in : FVT_lib/hal/convert_in  gain=10  offset=0
  VHAL_FLTurnLampC_mA : Outport
  wires:
  convert_in/1 -> VHAL_FLTurnLampC_mA/1
  UnitConverter/1 -> convert_in/1
  FLTurnLampC/1 -> UnitConverter/1

== system halin/HAL_IN/CAN4/ZONE_FR1/FLTurnLightWarning ==
  FLTurn_Light_Warning : Inport
  UnitConverter : DataTypeConversion  OutDataTypeStr=uint8
  VHAL_FLTurnLightWarning_flg : Outport
  wires:
  UnitConverter/1 -> VHAL_FLTurnLightWarning_flg/1
  FLTurn_Light_Warning/1 -> UnitConverter/1

== system halin/HAL_IN/CAN4/ZONE_FR1/FRTurnLPErr ==
  FRTurnLPErr : Inport
  UnitConverter : DataTypeConversion  OutDataTypeStr=uint8
  VHAL_FRTurnLPErr_flg : Outport
  wires:
  UnitConverter/1 -> VHAL_FRTurnLPErr_flg/1
  FRTurnLPErr/1 -> UnitConverter/1

== system halin/HAL_IN/CAN4/ZONE_FR1/FRTurnLampC ==
  FRTurnLampC : Inport
  UnitConverter : DataTypeConversion  OutDataTypeStr=uint8
  convert_in : FVT_lib/hal/convert_in  gain=10  offset=0
  VHAL_FRTurnLampC_mA : Outport
  wires:
  convert_in/1 -> VHAL_FRTurnLampC_mA/1
  UnitConverter/1 -> convert_in/1
  FRTurnLampC/1 -> UnitConverter/1

== system halin/HAL_IN/CAN4/ZONE_FR1/FRTurnLightWarning ==
  FRTurn_Light_Warning : Inport
  UnitConverter : DataTypeConversion  OutDataTypeStr=uint8
  VHAL_FRTurnLightWarning_flg : Outport
  wires:
  UnitConverter/1 -> VHAL_FRTurnLightWarning_flg/1
  FRTurn_Light_Warning/1 -> UnitConverter/1

== system halin/HAL_IN/CAN4/ZONE_FR1/FWiperAS ==
  FWiperAS : Inport
  UnitConverter : DataTypeConversion  OutDataTypeStr=uint8
  VHAL_FWiperAS_flg : Outport
  wires:
  UnitConverter/1 -> VHAL_FWiperAS_flg/1
  FWiperAS/1 -> UnitConverter/1

== system halin/HAL_IN/CAN4/ZONE_FR1/FWiperProtection ==
  FWiperProtection : Inport
  UnitConverter : DataTypeConversion  OutDataTypeStr=uint8
  VHAL_FWiperProtection_flg : Outport
  wires:
  UnitConverter/1 -> VHAL_FWiperProtection_flg/1
  FWiperProtection/1 -> UnitConverter/1

== system halin/HAL_IN/CAN4/ZONE_FR1/LADBHibeamIndication ==
  LADB_Hibeam_Indication : Inport
  UnitConverter : DataTypeConversion  OutDataTypeStr=uint8
  VHAL_LADBHibeamIndication_flg : Outport
  wires:
  UnitConverter/1 -> VHAL_LADBHibeamIndication_flg/1
  LADB_Hibeam_Indication/1 -> UnitConverter/1

== system halin/HAL_IN/CAN4/ZONE_FR1/LADBOperationStatus ==
  LADB_Operation_Status : Inport
  UnitConverter : DataTypeConversion  OutDataTypeStr=uint8
  VHAL_LADBOperationStatus_flg : Outport
  wires:
  UnitConverter/1 -> VHAL_LADBOperationStatus_flg/1
  LADB_Operation_Status/1 -> UnitConverter/1

== system halin/HAL_IN/CAN4/ZONE_FR1/LADBWarning ==
  LADB_Warning : Inport
  UnitConverter : DataTypeConversion  OutDataTypeStr=uint8
  VHAL_LADBWarning_flg : Outport
  wires:
  UnitConverter/1 -> VHAL_LADBWarning_flg/1
  LADB_Warning/1 -> UnitConverter/1

== system halin/HAL_IN/CAN4/ZONE_FR1/LAHBWarning ==
  LAHB_Warning : Inport
  UnitConverter : DataTypeConversion  OutDataTypeStr=uint8
  VHAL_LAHBWarning_flg : Outport
  wires:
  UnitConverter/1 -> VHAL_LAHBWarning_flg/1
  LAHB_Warning/1 -> UnitConverter/1

== system halin/HAL_IN/CAN4/ZONE_FR1/LDRLWarning ==
  LDRL_Warning : Inport
  UnitConverter : DataTypeConversion  OutDataTypeStr=uint8
  VHAL_LDRLWarning_flg : Outport
  wires:
  UnitConverter/1 -> VHAL_LDRLWarning_flg/1
  LDRL_Warning/1 -> UnitConverter/1

== system halin/HAL_IN/CAN4/ZONE_FR1/LLBWarning ==
  LLB_Warning : Inport
  UnitConverter : DataTypeConversion  OutDataTypeStr=uint8
  VHAL_LLBWarning_flg : Outport
  wires:
  UnitConverter/1 -> VHAL_LLBWarning_flg/1
  LLB_Warning/1 -> UnitConverter/1

== system halin/HAL_IN/CAN4/ZONE_FR1/LpositionLampWarning ==
  Lposition_Lamp_Warning : Inport
  UnitConverter : DataTypeConversion  OutDataTypeStr=uint8
  VHAL_LpositionLampWarning_flg : Outport
  wires:
  UnitConverter/1 -> VHAL_LpositionLampWarning_flg/1
  Lposition_Lamp_Warning/1 -> UnitConverter/1

== system halin/HAL_IN/CAN4/ZONE_FR1/RADBHibeamIndication ==
  RADB_Hibeam_Indication : Inport
  UnitConverter : DataTypeConversion  OutDataTypeStr=uint8
  VHAL_RADBHibeamIndication_flg : Outport
  wires:
  UnitConverter/1 -> VHAL_RADBHibeamIndication_flg/1
  RADB_Hibeam_Indication/1 -> UnitConverter/1

== system halin/HAL_IN/CAN4/ZONE_FR1/RADBOperationStatus ==
  RADB_Operation_Status : Inport
  UnitConverter : DataTypeConversion  OutDataTypeStr=uint8
  VHAL_RADBOperationStatus_flg : Outport
  wires:
  UnitConverter/1 -> VHAL_RADBOperationStatus_flg/1
  RADB_Operation_Status/1 -> UnitConverter/1

== system halin/HAL_IN/CAN4/ZONE_FR1/RADBWarning ==
  RADB_Warning : Inport
  UnitConverter : DataTypeConversion  OutDataTypeStr=uint8
  VHAL_RADBWarning_flg : Outport
  wires:
  UnitConverter/1 -> VHAL_RADBWarning_flg/1
  RADB_Warning/1 -> UnitConverter/1

== system halin/HAL_IN/CAN4/ZONE_FR1/RAHBWarning ==
  RAHB_Warning : Inport
  UnitConverter : DataTypeConversion  OutDataTypeStr=uint8
  VHAL_RAHBWarning_flg : Outport
  wires:
  UnitConverter/1 -> VHAL_RAHBWarning_flg/1
  RAHB_Warning/1 -> UnitConverter/1

== system halin/HAL_IN/CAN4/ZONE_FR1/RDRLWarning ==
  RDRL_Warning : Inport
  UnitConverter : DataTypeConversion  OutDataTypeStr=uint8
  VHAL_RDRLWarning_flg : Outport
  wires:
  UnitConverter/1 -> VHAL_RDRLWarning_flg/1
  RDRL_Warning/1 -> UnitConverter/1

== system halin/HAL_IN/CAN4/ZONE_FR1/RLBWarning ==
  RLB_Warning : Inport
  UnitConverter : DataTypeConversion  OutDataTypeStr=uint8
  VHAL_RLBWarning_flg : Outport
  wires:
  UnitConverter/1 -> VHAL_RLBWarning_flg/1
  RLB_Warning/1 -> UnitConverter/1

== system halin/HAL_IN/CAN4/ZONE_FR1/RpositionLampWarning ==
  Rposition_Lamp_Warning : Inport
  UnitConverter : DataTypeConversion  OutDataTypeStr=uint8
  VHAL_RpositionLampWarning_flg : Outport
  wires:
  UnitConverter/1 -> VHAL_RpositionLampWarning_flg/1
  Rposition_Lamp_Warning/1 -> UnitConverter/1

== system halin/HAL_IN/CAN4/ZONE_FR1/TrailerCheck ==
  TrailerCheck : Inport
  UnitConverter : DataTypeConversion  OutDataTypeStr=uint8
  VHAL_TrailerCheck_flg : Outport
  wires:
  UnitConverter/1 -> VHAL_TrailerCheck_flg/1
  TrailerCheck/1 -> UnitConverter/1

== system halin/HAL_IN/CAN4/ZONE_FR1/TrailerModeSta ==
  TrailerModeSta : Inport
  UnitConverter : DataTypeConversion  OutDataTypeStr=uint8
  VHAL_TrailerModeSta_enum : Outport
  wires:
  UnitConverter/1 -> VHAL_TrailerModeSta_enum/1
  TrailerModeSta/1 -> UnitConverter/1

== system halin/HAL_IN/CAN4/ZONE_FR1/ZFRBCMChargerDoorSWSta ==
  ZFR_BCM_ChargerDoorSW_Sta : Inport
  UnitConverter : DataTypeConversion  OutDataTypeStr=uint8
  VHAL_ZFRBCMChargerDoorSWSta_flg : Outport
  wires:
  UnitConverter/1 -> VHAL_ZFRBCMChargerDoorSWSta_flg/1
  ZFR_BCM_ChargerDoorSW_Sta/1 -> UnitConverter/1

== system halin/HAL_IN/CAN4/ZONE_FR1/ZFRBCMHRLTurnLPNormalSta ==
  ZFR_BCM_HRLTurnLPNormal_Sta : Inport
  UnitConverter : DataTypeConversion  OutDataTypeStr=uint8
  VHAL_ZFRBCMHRLTurnLPNormalSta_flg : Outport
  wires:
  UnitConverter/1 -> VHAL_ZFRBCMHRLTurnLPNormalSta_flg/1
  ZFR_BCM_HRLTurnLPNormal_Sta/1 -> UnitConverter/1

== system halin/HAL_IN/CAN4/ZONE_FR1/ZFRBCMHRRTurnLPHNormalSta ==
  ZFR_BCM_HRRTurnLPHNormal_Sta : Inport
  UnitConverter : DataTypeConversion  OutDataTypeStr=uint8
  VHAL_ZFRBCMHRRTurnLPHNormalSta_flg : Outport
  wires:
  UnitConverter/1 -> VHAL_ZFRBCMHRRTurnLPHNormalSta_flg/1
  ZFR_BCM_HRRTurnLPHNormal_Sta/1 -> UnitConverter/1

== system halin/HAL_IN/CAN4/ZONE_FR1/ZFRTHCMCLEVentActYSta ==
  ZFR_THCM_CLEVentActY_Sta : Inport
  UnitConverter : DataTypeConversion  OutDataTypeStr=uint8
  VHAL_ZFRTHCMCLEVentActYSta_pct : Outport
  wires:
  UnitConverter/1 -> VHAL_ZFRTHCMCLEVentActYSta_pct/1
  ZFR_THCM_CLEVentActY_Sta/1 -> UnitConverter/1

== system halin/HAL_IN/CAN4/ZONE_FR1/ZFRTHCMCREVentActYSta ==
  ZFR_THCM_CREVentActY_Sta : Inport
  UnitConverter : DataTypeConversion  OutDataTypeStr=uint8
  VHAL_ZFRTHCMCREVentActYSta_pct : Outport
  wires:
  UnitConverter/1 -> VHAL_ZFRTHCMCREVentActYSta_pct/1
  ZFR_THCM_CREVentActY_Sta/1 -> UnitConverter/1

== system halin/HAL_IN/CAN4/ZONE_FR1/ZFRTHCMLEVentActYSta ==
  ZFR_THCM_LEVentActY_Sta : Inport
  UnitConverter : DataTypeConversion  OutDataTypeStr=uint8
  VHAL_ZFRTHCMLEVentActYSta_pct : Outport
  wires:
  UnitConverter/1 -> VHAL_ZFRTHCMLEVentActYSta_pct/1
  ZFR_THCM_LEVentActY_Sta/1 -> UnitConverter/1

== system halin/HAL_IN/CAN4/ZONE_FR1/ZFRTHCMREVentActYSta ==
  ZFR_THCM_REVentActY_Sta : Inport
  UnitConverter : DataTypeConversion  OutDataTypeStr=uint8
  VHAL_ZFRTHCMREVentActYSta_pct : Outport
  wires:
  UnitConverter/1 -> VHAL_ZFRTHCMREVentActYSta_pct/1
  ZFR_THCM_REVentActY_Sta/1 -> UnitConverter/1

== system halin/HAL_IN/CAN4/ZONE_FR_VCU/AGSErr ==
  AGS_Err : Inport
  UnitConverter : DataTypeConversion  OutDataTypeStr=uint8
  VHAL_AGSErr_enum : Outport
  wires:
  UnitConverter/1 -> VHAL_AGSErr_enum/1
  AGS_Err/1 -> UnitConverter/1

== system halin/HAL_IN/CAN4/ZONE_FR_VCU/BatInTemp ==
  Bat_In_Temp : Inport
  UnitConverter : DataTypeConversion  OutDataTypeStr=uint8
  convert_in : FVT_lib/hal/convert_in  gain=0.5  offset=-40
  VHAL_BatInTemp_C : Outport
  wires:
  convert_in/1 -> VHAL_BatInTemp_C/1
  UnitConverter/1 -> convert_in/1
  Bat_In_Temp/1 -> UnitConverter/1

== system halin/HAL_IN/CAN4/ZONE_FR_VCU/BatInTempErr ==
  Bat_In_Temp_Err : Inport
  UnitConverter : DataTypeConversion  OutDataTypeStr=uint8
  VHAL_BatInTempErr_enum : Outport
  wires:
  UnitConverter/1 -> VHAL_BatInTempErr_enum/1
  Bat_In_Temp_Err/1 -> UnitConverter/1

== system halin/HAL_IN/CAN4/ZONE_FR_VCU/BatOutTemp ==
  Bat_Out_Temp : Inport
  UnitConverter : DataTypeConversion  OutDataTypeStr=uint8
  convert_in : FVT_lib/hal/convert_in  gain=0.5  offset=-40
  VHAL_BatOutTemp_C : Outport
  wires:
  convert_in/1 -> VHAL_BatOutTemp_C/1
  UnitConverter/1 -> convert_in/1
  Bat_Out_Temp/1 -> UnitConverter/1

== system halin/HAL_IN/CAN4/ZONE_FR_VCU/COMPErr ==
  COMP_Err : Inport
  UnitConverter : DataTypeConversion  OutDataTypeStr=uint8
  VHAL_COMPErr_enum : Outport
  wires:
  UnitConverter/1 -> VHAL_COMPErr_enum/1
  COMP_Err/1 -> UnitConverter/1

== system halin/HAL_IN/CAN4/ZONE_FR_VCU/EACProtectEnable ==
  EACProtectEnable : Inport
  UnitConverter : DataTypeConversion  OutDataTypeStr=uint8
  VHAL_EACProtectEnable_enum : Outport
  wires:
  UnitConverter/1 -> VHAL_EACProtectEnable_enum/1
  EACProtectEnable/1 -> UnitConverter/1

== system halin/HAL_IN/CAN4/ZONE_FR_VCU/EWP3Err ==
  EWP3_Err : Inport
  UnitConverter : DataTypeConversion  OutDataTypeStr=uint8
  VHAL_EWP3Err_enum : Outport
  wires:
  UnitConverter/1 -> VHAL_EWP3Err_enum/1
  EWP3_Err/1 -> UnitConverter/1

== system halin/HAL_IN/CAN4/ZONE_FR_VCU/EXV1Err ==
  EXV1_Err : Inport
  UnitConverter : DataTypeConversion  OutDataTypeStr=uint8
  VHAL_EXV1Err_enum : Outport
  wires:
  UnitConverter/1 -> VHAL_EXV1Err_enum/1
  EXV1_Err/1 -> UnitConverter/1

== system halin/HAL_IN/CAN4/ZONE_FR_VCU/EXV2Err ==
  EXV2_Err : Inport
  UnitConverter : DataTypeConversion  OutDataTypeStr=uint8
  VHAL_EXV2Err_enum : Outport
  wires:
  UnitConverter/1 -> VHAL_EXV2Err_enum/1
  EXV2_Err/1 -> UnitConverter/1

== system halin/HAL_IN/CAN4/ZONE_FR_VCU/FanErr ==
  Fan_Err : Inport
  UnitConverter : DataTypeConversion  OutDataTypeStr=uint8
  VHAL_FanErr_enum : Outport
  wires:
  UnitConverter/1 -> VHAL_FanErr_enum/1
  Fan_Err/1 -> UnitConverter/1

== system halin/HAL_IN/CAN4/ZONE_FR_VCU/FrPMMLimpHomeActReq ==
  FrPMMLimpHomeActReq : Inport
  UnitConverter : DataTypeConversion  OutDataTypeStr=uint8
  VHAL_FrPMMLimpHomeActReq_flg : Outport
  wires:
  UnitConverter/1 -> VHAL_FrPMMLimpHomeActReq_flg/1
  FrPMMLimpHomeActReq/1 -> UnitConverter/1

== system halin/HAL_IN/CAN4/ZONE_FR_VCU/MotorInTemp ==
  Motor_In_Temp : Inport
  UnitConverter : DataTypeConversion  OutDataTypeStr=uint8
  convert_in : FVT_lib/hal/convert_in  gain=0.5  offset=-40
  VHAL_MotorInTemp_C : Outport
  wires:
  convert_in/1 -> VHAL_MotorInTemp_C/1
  UnitConverter/1 -> convert_in/1
  Motor_In_Temp/1 -> UnitConverter/1

== system halin/HAL_IN/CAN4/ZONE_FR_VCU/MotorInTempErr ==
  Motor_In_Temp_Err : Inport
  UnitConverter : DataTypeConversion  OutDataTypeStr=uint8
  VHAL_MotorInTempErr_enum : Outport
  wires:
  UnitConverter/1 -> VHAL_MotorInTempErr_enum/1
  Motor_In_Temp_Err/1 -> UnitConverter/1

== system halin/HAL_IN/CAN4/ZONE_FR_VCU/MotorOutTemp ==
  Motor_Out_Temp : Inport
  UnitConverter : DataTypeConversion  OutDataTypeStr=uint8
  convert_in : FVT_lib/hal/convert_in  gain=0.5  offset=-40
  VHAL_MotorOutTemp_C : Outport
  wires:
  convert_in/1 -> VHAL_MotorOutTemp_C/1
  UnitConverter/1 -> convert_in/1
  Motor_Out_Temp/1 -> UnitConverter/1

== system halin/HAL_IN/CAN4/ZONE_FR_VCU/MotorOutTempErr ==
  Motor_Out_Temp_Err : Inport
  UnitConverter : DataTypeConversion  OutDataTypeStr=uint8
  VHAL_MotorOutTempErr_enum : Outport
  wires:
  UnitConverter/1 -> VHAL_MotorOutTempErr_enum/1
  Motor_Out_Temp_Err/1 -> UnitConverter/1

== system halin/HAL_IN/CAN4/ZONE_FR_VCU/PTHighP ==
  PT_High_P : Inport
  UnitConverter : DataTypeConversion  OutDataTypeStr=uint16
  VHAL_PTHighP_KPa : Outport
  wires:
  UnitConverter/1 -> VHAL_PTHighP_KPa/1
  PT_High_P/1 -> UnitConverter/1

== system halin/HAL_IN/CAN4/ZONE_FR_VCU/PTHighPErr ==
  PT_High_P_Err : Inport
  UnitConverter : DataTypeConversion  OutDataTypeStr=uint8
  VHAL_PTHighPErr_enum : Outport
  wires:
  UnitConverter/1 -> VHAL_PTHighPErr_enum/1
  PT_High_P_Err/1 -> UnitConverter/1

== system halin/HAL_IN/CAN4/ZONE_FR_VCU/PTHighTact ==
  PT_High_Tact : Inport
  UnitConverter : DataTypeConversion  OutDataTypeStr=uint8
  convert_in : FVT_lib/hal/convert_in  gain=1  offset=-40
  VHAL_PTHighTact_C : Outport
  wires:
  convert_in/1 -> VHAL_PTHighTact_C/1
  UnitConverter/1 -> convert_in/1
  PT_High_Tact/1 -> UnitConverter/1

== system halin/HAL_IN/CAN4/ZONE_FR_VCU/PTHighTactErr ==
  PT_High_Tact_Err : Inport
  UnitConverter : DataTypeConversion  OutDataTypeStr=uint8
  VHAL_PTHighTactErr_enum : Outport
  wires:
  UnitConverter/1 -> VHAL_PTHighTactErr_enum/1
  PT_High_Tact_Err/1 -> UnitConverter/1

== system halin/HAL_IN/CAN4/ZONE_FR_VCU/PTLowP1 ==
  PT_Low_P1 : Inport
  UnitConverter : DataTypeConversion  OutDataTypeStr=uint16
  VHAL_PTLowP1_KPa : Outport
  wires:
  UnitConverter/1 -> VHAL_PTLowP1_KPa/1
  PT_Low_P1/1 -> UnitConverter/1

== system halin/HAL_IN/CAN4/ZONE_FR_VCU/PTLowP1Err ==
  PT_Low_P1_Err : Inport
  UnitConverter : DataTypeConversion  OutDataTypeStr=uint8
  VHAL_PTLowP1Err_enum : Outport
  wires:
  UnitConverter/1 -> VHAL_PTLowP1Err_enum/1
  PT_Low_P1_Err/1 -> UnitConverter/1

== system halin/HAL_IN/CAN4/ZONE_FR_VCU/PTLowP2 ==
  PT_Low_P2 : Inport
  UnitConverter : DataTypeConversion  OutDataTypeStr=uint16
  VHAL_PTLowP2_KPa : Outport
  wires:
  UnitConverter/1 -> VHAL_PTLowP2_KPa/1
  PT_Low_P2/1 -> UnitConverter/1

== system halin/HAL_IN/CAN4/ZONE_FR_VCU/PTLowP2Err ==
  PT_Low_P2_Err : Inport
  UnitConverter : DataTypeConversion  OutDataTypeStr=uint8
  VHAL_PTLowP2Err_enum : Outport
  wires:
  UnitConverter/1 -> VHAL_PTLowP2Err_enum/1
  PT_Low_P2_Err/1 -> UnitConverter/1
